simulink model "chap4_3sim"  (Simulink 7.7)
settings: Solver=ode45  StartTime=0.0  StopTime=3  RelTol=1e-3
libraries: fuzblock x1
settings Model: Creator=ljk  LastModifiedBy=ljk
settings DataIOCC: SignalLoggingName=sigsOut
settings DebuggingCC: SaveWithParameterizedLinksMsg=none  SignalResolutionControl=TryResolveAllWithWarning  SolverPrmCheckMsg=none  MultiTaskDSMMsg=warning  MultiTaskCondExecSysMsg=none  StrictBusMsg=None
settings HardwareCC: TargetUnknown=on
settings RTWCC: IncludeERTFirstTime=on

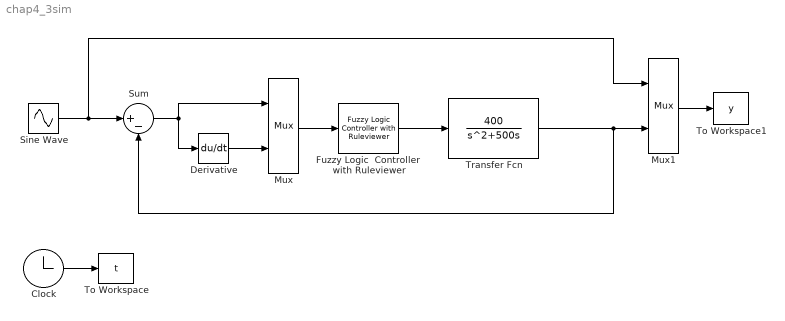
== system chap4_3sim ==
  Clock : Clock
      settings: Decimation=10
  Derivative : Derivative
  Fuzzy Logic  Controller  with Ruleviewer : fuzblock/Fuzzy Logic  Controller  with Ruleviewer  SystemSampleTime=-1  fismatrix=a2  Ts=2
      link override Fuzzy Logic Controller: fis=a2
  Mux : Mux  Inputs=2
  Mux1 : Mux  Inputs=2
  Sine Wave : Sin  Amplitude=0.5  Frequency=10  SampleTime=0
  Sum : Sum  Inputs=|+-  SaturateOnIntegerOverflow=on  InputSameDT=on  OutDataTypeStr=Inherit: Same as first input
  To Workspace : ToWorkspace  VariableName=t  SampleTime=-1  SaveFormat=Array
  To Workspace1 : ToWorkspace  VariableName=y  SampleTime=-1  SaveFormat=Array
  Transfer Fcn : TransferFcn  Numerator=[400]  Denominator=[1 500 0]
  wires:
  Mux/1 -> Fuzzy Logic  Controller  with Ruleviewer/1
  Derivative/1 -> Mux/2
  Sum/1 -> Mux/1, Derivative/1
  Sine Wave/1 -> Sum/1, Mux1/1
  Mux1/1 -> To Workspace1/1
  Fuzzy Logic  Controller  with Ruleviewer/1 -> Transfer Fcn/1
  Transfer Fcn/1 -> Mux1/2, Sum/2
  Clock/1 -> To Workspace/1
